simulink model "UserVehicle_RTW"  (R2022b)
settings: Solver=ode1  StartTime=0.0  StopTime=inf  FixedStep=0.001  RelTol=1e-3
PreLoadFcn:
  | vehicle = 'Car'; if ~length(which('cmself')), cmenv; end
  | UserVehicle_RTW_bus
  | UserVehicle_RTW_params
InitFcn:
  | vehicle = 'Car'; if ~length(which('cmself')), cmenv; end
  | UserVehicle_RTW_bus
values from neighbouring files (symbols this model uses):
  Car_Bdy1_mass = 650.0    (= 650)    [SingleTrack_RTW_params.m]    (also in UserVehicle_RTW_params.m)
  Car_Steering_i = 10.0    (= 10)    [SingleTrack_RTW_params.m]    (also in UserVehicle_RTW_params.m)
  Car_WhlBaseF = 1.5    [SingleTrack_RTW_params.m]    (also in UserVehicle_RTW_params.m)
  Car_WhlBaseR = -1.5    [SingleTrack_RTW_params.m]    (also in UserVehicle_RTW_params.m)
libraries: CarMaker4SL x77
(part 2 of 3)

== system UserVehicle_RTW/SingleTrack_Out/Subsystem1 ==
  In1 : Inport
  Bus Creator : BusCreator  Inputs=3
  foo_Input_Selector1 : BusSelector  OutputSignals=Vhcl v,Vhcl Distance,Vhcl sRoad,Vhcl Hitch_Pos x,Vhcl Hitch_Pos y,Vhcl Hitch_Pos z,Vhcl Roll,Vhcl RollVel,Vhcl RollAcc,Vhcl Pitch,Vhcl PitchVel,Vhcl PitchAcc,Vhcl Yaw,Vhcl YawRate,Vhcl YawAcc
  Out1 : Outport  VectorParamsAs1DForOutWhenUnconnected=off
  Out2 : Outport  Port=2  VectorParamsAs1DForOutWhenUnconnected=off
  Out3 : Outport  Port=3  VectorParamsAs1DForOutWhenUnconnected=off
  Out6 : Outport  Port=4  VectorParamsAs1DForOutWhenUnconnected=off
  Out7 : Outport  Port=5  VectorParamsAs1DForOutWhenUnconnected=off
  Out8 : Outport  Port=6  VectorParamsAs1DForOutWhenUnconnected=off
  Out9 : Outport  Port=7  VectorParamsAs1DForOutWhenUnconnected=off
  Out10 : Outport  Port=8  VectorParamsAs1DForOutWhenUnconnected=off
  Out11 : Outport  Port=9  VectorParamsAs1DForOutWhenUnconnected=off
  Out12 : Outport  Port=10  VectorParamsAs1DForOutWhenUnconnected=off
  Out13 : Outport  Port=11  VectorParamsAs1DForOutWhenUnconnected=off
  Out14 : Outport  Port=12  VectorParamsAs1DForOutWhenUnconnected=off
  Out15 : Outport  Port=13  VectorParamsAs1DForOutWhenUnconnected=off
  wires:
  foo_Input_Selector1/4 -> Bus Creator/1  "<Vhcl Hitch_Pos x>"
  foo_Input_Selector1/5 -> Bus Creator/2  "<Vhcl Hitch_Pos y>"
  foo_Input_Selector1/6 -> Bus Creator/3  "<Vhcl Hitch_Pos z>"
  foo_Input_Selector1/1 -> Out1/1  "<Vhcl v>"
  foo_Input_Selector1/2 -> Out2/1  "<Vhcl Distance>"
  foo_Input_Selector1/3 -> Out3/1  "<Vhcl sRoad>"
  Bus Creator/1 -> Out6/1
  foo_Input_Selector1/7 -> Out7/1  "<Vhcl Roll>"
  foo_Input_Selector1/8 -> Out8/1  "<Vhcl RollVel>"
  foo_Input_Selector1/9 -> Out9/1  "<Vhcl RollAcc>"
  foo_Input_Selector1/10 -> Out10/1  "<Vhcl Pitch>"
  foo_Input_Selector1/11 -> Out11/1  "<Vhcl PitchVel>"
  foo_Input_Selector1/12 -> Out12/1  "<Vhcl PitchAcc>"
  foo_Input_Selector1/13 -> Out13/1  "<Vhcl Yaw>"
  foo_Input_Selector1/14 -> Out14/1  "<Vhcl YawRate>"
  foo_Input_Selector1/15 -> Out15/1  "<Vhcl YawAcc>"
  In1/1 -> foo_Input_Selector1/1

== system UserVehicle_RTW/SingleTrack_Out/Subsystem2 ==
  In1 : Inport
  Bus Creator : BusCreator  Inputs=3
  Bus Creator1 : BusCreator  Inputs=3
  foo_Input_Selector3 : BusSelector  OutputSignals=Vhcl Wheel FL t x,Vhcl Wheel FL t y,Vhcl Wheel FL t z,Vhcl Wheel FL r_zxy x,Vhcl Wheel FL r_zxy y,Vhcl Wheel FL r_zxy z,Vhcl Wheel FL Fx,Vhcl Wheel FL Fy,Vhcl Wheel FL Fz,Vhcl Wheel FL vBelt,Vhcl Wheel FL LongSlip,Vhcl Wheel FL SideSlip,Vhcl Wheel FL Trq_T2W,Vhcl Wheel FL Trq_WhlBearing
  Out1 : Outport  VectorParamsAs1DForOutWhenUnconnected=off
  Out2 : Outport  Port=2  VectorParamsAs1DForOutWhenUnconnected=off
  Out3 : Outport  Port=3  VectorParamsAs1DForOutWhenUnconnected=off
  Out4 : Outport  Port=4  VectorParamsAs1DForOutWhenUnconnected=off
  Out5 : Outport  Port=5  VectorParamsAs1DForOutWhenUnconnected=off
  Out6 : Outport  Port=6  VectorParamsAs1DForOutWhenUnconnected=off
  Out7 : Outport  Port=7  VectorParamsAs1DForOutWhenUnconnected=off
  Out8 : Outport  Port=8  VectorParamsAs1DForOutWhenUnconnected=off
  Out9 : Outport  Port=9  VectorParamsAs1DForOutWhenUnconnected=off
  Out10 : Outport  Port=10  VectorParamsAs1DForOutWhenUnconnected=off
  wires:
  foo_Input_Selector3/1 -> Bus Creator1/1  "<Vhcl Wheel FL t x>"
  foo_Input_Selector3/2 -> Bus Creator1/2  "<Vhcl Wheel FL t y>"
  foo_Input_Selector3/3 -> Bus Creator1/3  "<Vhcl Wheel FL t z>"
  foo_Input_Selector3/4 -> Bus Creator/1  "<Vhcl Wheel FL r_zxy x>"
  foo_Input_Selector3/5 -> Bus Creator/2  "<Vhcl Wheel FL r_zxy y>"
  foo_Input_Selector3/6 -> Bus Creator/3  "<Vhcl Wheel FL r_zxy z>"
  Bus Creator1/1 -> Out1/1
  Bus Creator/1 -> Out2/1
  foo_Input_Selector3/7 -> Out3/1  "<Vhcl Wheel FL Fx>"
  In1/1 -> foo_Input_Selector3/1
  foo_Input_Selector3/8 -> Out4/1  "<Vhcl Wheel FL Fy>"
  foo_Input_Selector3/9 -> Out5/1  "<Vhcl Wheel FL Fz>"
  foo_Input_Selector3/10 -> Out6/1  "<Vhcl Wheel FL vBelt>"
  foo_Input_Selector3/11 -> Out7/1  "<Vhcl Wheel FL LongSlip>"
  foo_Input_Selector3/12 -> Out8/1  "<Vhcl Wheel FL SideSlip>"
  foo_Input_Selector3/13 -> Out9/1  "<Vhcl Wheel FL Trq_T2W>"
  foo_Input_Selector3/14 -> Out10/1  "<Vhcl Wheel FL Trq_WhlBearing>"

== system UserVehicle_RTW/SingleTrack_Out/Subsystem3 ==
  In1 : Inport
  Bus Creator : BusCreator  Inputs=3
  Bus Creator1 : BusCreator  Inputs=3
  foo_Input_Selector3 : BusSelector  OutputSignals=Vhcl Wheel FR t x,Vhcl Wheel FR t y,Vhcl Wheel FR t z,Vhcl Wheel FR r_zxy x,Vhcl Wheel FR r_zxy y,Vhcl Wheel FR r_zxy z,Vhcl Wheel FR Fx,Vhcl Wheel FR Fy,Vhcl Wheel FR Fz,Vhcl Wheel FR vBelt,Vhcl Wheel FR LongSlip,Vhcl Wheel FR SideSlip,Vhcl Wheel FR Trq_T2W,Vhcl Wheel FR Trq_WhlBearing
  Out1 : Outport  VectorParamsAs1DForOutWhenUnconnected=off
  Out2 : Outport  Port=2  VectorParamsAs1DForOutWhenUnconnected=off
  Out3 : Outport  Port=3  VectorParamsAs1DForOutWhenUnconnected=off
  Out4 : Outport  Port=4  VectorParamsAs1DForOutWhenUnconnected=off
  Out5 : Outport  Port=5  VectorParamsAs1DForOutWhenUnconnected=off
  Out6 : Outport  Port=6  VectorParamsAs1DForOutWhenUnconnected=off
  Out7 : Outport  Port=7  VectorParamsAs1DForOutWhenUnconnected=off
  Out8 : Outport  Port=8  VectorParamsAs1DForOutWhenUnconnected=off
  Out9 : Outport  Port=9  VectorParamsAs1DForOutWhenUnconnected=off
  Out10 : Outport  Port=10  VectorParamsAs1DForOutWhenUnconnected=off
  wires:
  foo_Input_Selector3/1 -> Bus Creator/1  "<Vhcl Wheel FR t x>"
  foo_Input_Selector3/2 -> Bus Creator/2  "<Vhcl Wheel FR t y>"
  foo_Input_Selector3/3 -> Bus Creator/3  "<Vhcl Wheel FR t z>"
  foo_Input_Selector3/4 -> Bus Creator1/1  "<Vhcl Wheel FR r_zxy x>"
  foo_Input_Selector3/5 -> Bus Creator1/2  "<Vhcl Wheel FR r_zxy y>"
  foo_Input_Selector3/6 -> Bus Creator1/3  "<Vhcl Wheel FR r_zxy z>"
  Bus Creator/1 -> Out1/1
  Bus Creator1/1 -> Out2/1
  foo_Input_Selector3/7 -> Out3/1  "<Vhcl Wheel FR Fx>"
  In1/1 -> foo_Input_Selector3/1
  foo_Input_Selector3/8 -> Out4/1  "<Vhcl Wheel FR Fy>"
  foo_Input_Selector3/9 -> Out5/1  "<Vhcl Wheel FR Fz>"
  foo_Input_Selector3/10 -> Out6/1  "<Vhcl Wheel FR vBelt>"
  foo_Input_Selector3/11 -> Out7/1  "<Vhcl Wheel FR LongSlip>"
  foo_Input_Selector3/12 -> Out8/1  "<Vhcl Wheel FR SideSlip>"
  foo_Input_Selector3/13 -> Out9/1  "<Vhcl Wheel FR Trq_T2W>"
  foo_Input_Selector3/14 -> Out10/1  "<Vhcl Wheel FR Trq_WhlBearing>"

== system UserVehicle_RTW/SingleTrack_Out/Subsystem4 ==
  In1 : Inport
  Bus Creator : BusCreator  Inputs=3
  Bus Creator1 : BusCreator  Inputs=3
  foo_Input_Selector3 : BusSelector  OutputSignals=Vhcl Wheel RL t x,Vhcl Wheel RL t y,Vhcl Wheel RL t z,Vhcl Wheel RL r_zxy x,Vhcl Wheel RL r_zxy y,Vhcl Wheel RL r_zxy z,Vhcl Wheel RL Fx,Vhcl Wheel RL Fy,Vhcl Wheel RL Fz,Vhcl Wheel RL vBelt,Vhcl Wheel RL LongSlip,Vhcl Wheel RL SideSlip,Vhcl Wheel RL Trq_T2W,Vhcl Wheel RL Trq_WhlBearing
  Out1 : Outport  VectorParamsAs1DForOutWhenUnconnected=off
  Out2 : Outport  Port=2  VectorParamsAs1DForOutWhenUnconnected=off
  Out3 : Outport  Port=3  VectorParamsAs1DForOutWhenUnconnected=off
  Out4 : Outport  Port=4  VectorParamsAs1DForOutWhenUnconnected=off
  Out5 : Outport  Port=5  VectorParamsAs1DForOutWhenUnconnected=off
  Out6 : Outport  Port=6  VectorParamsAs1DForOutWhenUnconnected=off
  Out7 : Outport  Port=7  VectorParamsAs1DForOutWhenUnconnected=off
  Out8 : Outport  Port=8  VectorParamsAs1DForOutWhenUnconnected=off
  Out9 : Outport  Port=9  VectorParamsAs1DForOutWhenUnconnected=off
  Out10 : Outport  Port=10  VectorParamsAs1DForOutWhenUnconnected=off
  wires:
  foo_Input_Selector3/1 -> Bus Creator/1  "<Vhcl Wheel RL t x>"
  foo_Input_Selector3/2 -> Bus Creator/2  "<Vhcl Wheel RL t y>"
  foo_Input_Selector3/3 -> Bus Creator/3  "<Vhcl Wheel RL t z>"
  foo_Input_Selector3/4 -> Bus Creator1/1  "<Vhcl Wheel RL r_zxy x>"
  foo_Input_Selector3/5 -> Bus Creator1/2  "<Vhcl Wheel RL r_zxy y>"
  foo_Input_Selector3/6 -> Bus Creator1/3  "<Vhcl Wheel RL r_zxy z>"
  Bus Creator/1 -> Out1/1
  Bus Creator1/1 -> Out2/1
  foo_Input_Selector3/7 -> Out3/1  "<Vhcl Wheel RL Fx>"
  In1/1 -> foo_Input_Selector3/1
  foo_Input_Selector3/8 -> Out4/1  "<Vhcl Wheel RL Fy>"
  foo_Input_Selector3/9 -> Out5/1  "<Vhcl Wheel RL Fz>"
  foo_Input_Selector3/10 -> Out6/1  "<Vhcl Wheel RL vBelt>"
  foo_Input_Selector3/11 -> Out7/1  "<Vhcl Wheel RL LongSlip>"
  foo_Input_Selector3/12 -> Out8/1  "<Vhcl Wheel RL SideSlip>"
  foo_Input_Selector3/13 -> Out9/1  "<Vhcl Wheel RL Trq_T2W>"
  foo_Input_Selector3/14 -> Out10/1  "<Vhcl Wheel RL Trq_WhlBearing>"

== system UserVehicle_RTW/SingleTrack_Out/Subsystem5 ==
  In1 : Inport
  Bus Creator : BusCreator  Inputs=3
  Bus Creator1 : BusCreator  Inputs=3
  foo_Input_Selector3 : BusSelector  OutputSignals=Vhcl Wheel RR t x,Vhcl Wheel RR t y,Vhcl Wheel RR t z,Vhcl Wheel RR r_zxy x,Vhcl Wheel RR r_zxy y,Vhcl Wheel RR r_zxy z,Vhcl Wheel RR Fx,Vhcl Wheel RR Fy,Vhcl Wheel RR Fz,Vhcl Wheel RR vBelt,Vhcl Wheel RR LongSlip,Vhcl Wheel RR SideSlip,Vhcl Wheel RR Trq_T2W,Vhcl Wheel RR Trq_WhlBearing
  Out1 : Outport  VectorParamsAs1DForOutWhenUnconnected=off
  Out2 : Outport  Port=2  VectorParamsAs1DForOutWhenUnconnected=off
  Out3 : Outport  Port=3  VectorParamsAs1DForOutWhenUnconnected=off
  Out4 : Outport  Port=4  VectorParamsAs1DForOutWhenUnconnected=off
  Out5 : Outport  Port=5  VectorParamsAs1DForOutWhenUnconnected=off
  Out6 : Outport  Port=6  VectorParamsAs1DForOutWhenUnconnected=off
  Out7 : Outport  Port=7  VectorParamsAs1DForOutWhenUnconnected=off
  Out8 : Outport  Port=8  VectorParamsAs1DForOutWhenUnconnected=off
  Out9 : Outport  Port=9  VectorParamsAs1DForOutWhenUnconnected=off
  Out10 : Outport  Port=10  VectorParamsAs1DForOutWhenUnconnected=off
  wires:
  foo_Input_Selector3/1 -> Bus Creator/1  "<Vhcl Wheel RR t x>"
  foo_Input_Selector3/2 -> Bus Creator/2  "<Vhcl Wheel RR t y>"
  foo_Input_Selector3/3 -> Bus Creator/3  "<Vhcl Wheel RR t z>"
  foo_Input_Selector3/4 -> Bus Creator1/1  "<Vhcl Wheel RR r_zxy x>"
  foo_Input_Selector3/5 -> Bus Creator1/2  "<Vhcl Wheel RR r_zxy y>"
  foo_Input_Selector3/6 -> Bus Creator1/3  "<Vhcl Wheel RR r_zxy z>"
  Bus Creator/1 -> Out1/1
  Bus Creator1/1 -> Out2/1
  foo_Input_Selector3/7 -> Out3/1  "<Vhcl Wheel RR Fx>"
  In1/1 -> foo_Input_Selector3/1
  foo_Input_Selector3/8 -> Out4/1  "<Vhcl Wheel RR Fy>"
  foo_Input_Selector3/9 -> Out5/1  "<Vhcl Wheel RR Fz>"
  foo_Input_Selector3/10 -> Out6/1  "<Vhcl Wheel RR vBelt>"
  foo_Input_Selector3/11 -> Out7/1  "<Vhcl Wheel RR LongSlip>"
  foo_Input_Selector3/12 -> Out8/1  "<Vhcl Wheel RR SideSlip>"
  foo_Input_Selector3/13 -> Out9/1  "<Vhcl Wheel RR Trq_T2W>"
  foo_Input_Selector3/14 -> Out10/1  "<Vhcl Wheel RR Trq_WhlBearing>"

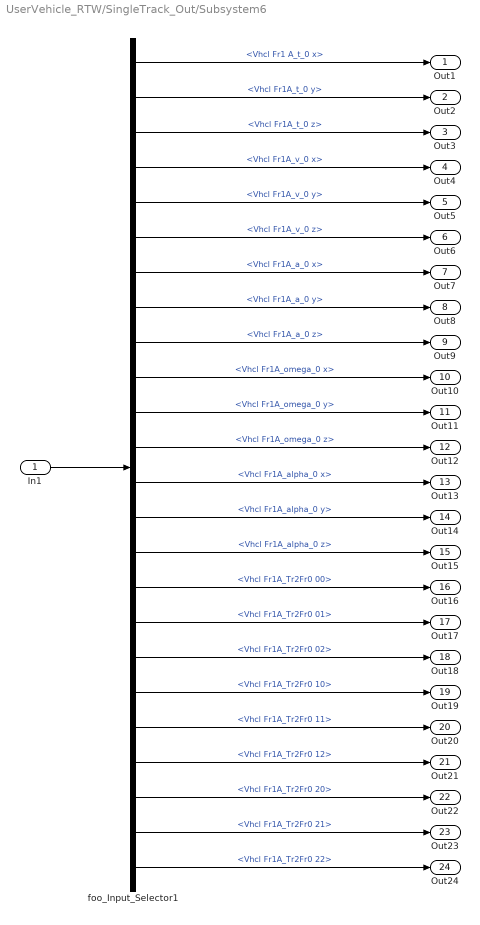
== system UserVehicle_RTW/SingleTrack_Out/Subsystem6 ==
  In1 : Inport
  foo_Input_Selector1 : BusSelector  OutputSignals=Vhcl Fr1 A_t_0 x,Vhcl Fr1A_t_0 y,Vhcl Fr1A_t_0 z,Vhcl Fr1A_v_0 x,Vhcl Fr1A_v_0 y,Vhcl Fr1A_v_0 z,Vhcl Fr1A_a_0 x,Vhcl Fr1A_a_0 y,Vhcl Fr1A_a_0 z,Vhcl Fr1A_omega_0 x,Vhcl Fr1A_omega_0 y,Vhcl Fr1A_omega_0 z,Vhcl Fr1A_alpha_0 x,Vhcl Fr1A_alpha_0 y,Vhcl Fr1A_alpha_0 z,Vhcl Fr1A_Tr2Fr0 00,Vhcl Fr1A_Tr2Fr0 01,Vhcl Fr1A_Tr2Fr0 02,Vhcl Fr1A_Tr2Fr0 10,Vhcl Fr1A_Tr2Fr0 11,Vhcl Fr1A_Tr2Fr0 12,Vhcl Fr1A_Tr2Fr0 20,Vhcl Fr1A_Tr2Fr0 21,Vhcl Fr1A_Tr2Fr0 22
  Out1 : Outport  VectorParamsAs1DForOutWhenUnconnected=off
  Out2 : Outport  Port=2  VectorParamsAs1DForOutWhenUnconnected=off
  Out3 : Outport  Port=3  VectorParamsAs1DForOutWhenUnconnected=off
  Out4 : Outport  Port=4  VectorParamsAs1DForOutWhenUnconnected=off
  Out5 : Outport  Port=5  VectorParamsAs1DForOutWhenUnconnected=off
  Out6 : Outport  Port=6  VectorParamsAs1DForOutWhenUnconnected=off
  Out7 : Outport  Port=7  VectorParamsAs1DForOutWhenUnconnected=off
  Out8 : Outport  Port=8  VectorParamsAs1DForOutWhenUnconnected=off
  Out9 : Outport  Port=9  VectorParamsAs1DForOutWhenUnconnected=off
  Out10 : Outport  Port=10  VectorParamsAs1DForOutWhenUnconnected=off
  Out11 : Outport  Port=11  VectorParamsAs1DForOutWhenUnconnected=off
  Out12 : Outport  Port=12  VectorParamsAs1DForOutWhenUnconnected=off
  Out13 : Outport  Port=13  VectorParamsAs1DForOutWhenUnconnected=off
  Out14 : Outport  Port=14  VectorParamsAs1DForOutWhenUnconnected=off
  Out15 : Outport  Port=15  VectorParamsAs1DForOutWhenUnconnected=off
  Out16 : Outport  Port=16  VectorParamsAs1DForOutWhenUnconnected=off
  Out17 : Outport  Port=17  VectorParamsAs1DForOutWhenUnconnected=off
  Out18 : Outport  Port=18  VectorParamsAs1DForOutWhenUnconnected=off
  Out19 : Outport  Port=19  VectorParamsAs1DForOutWhenUnconnected=off
  Out20 : Outport  Port=20  VectorParamsAs1DForOutWhenUnconnected=off
  Out21 : Outport  Port=21  VectorParamsAs1DForOutWhenUnconnected=off
  Out22 : Outport  Port=22  VectorParamsAs1DForOutWhenUnconnected=off
  Out23 : Outport  Port=23  VectorParamsAs1DForOutWhenUnconnected=off
  Out24 : Outport  Port=24  VectorParamsAs1DForOutWhenUnconnected=off
  wires:
  foo_Input_Selector1/24 -> Out24/1  "<Vhcl Fr1A_Tr2Fr0 22>"
  foo_Input_Selector1/23 -> Out23/1  "<Vhcl Fr1A_Tr2Fr0 21>"
  foo_Input_Selector1/22 -> Out22/1  "<Vhcl Fr1A_Tr2Fr0 20>"
  foo_Input_Selector1/21 -> Out21/1  "<Vhcl Fr1A_Tr2Fr0 12>"
  foo_Input_Selector1/20 -> Out20/1  "<Vhcl Fr1A_Tr2Fr0 11>"
  foo_Input_Selector1/19 -> Out19/1  "<Vhcl Fr1A_Tr2Fr0 10>"
  foo_Input_Selector1/18 -> Out18/1  "<Vhcl Fr1A_Tr2Fr0 02>"
  foo_Input_Selector1/17 -> Out17/1  "<Vhcl Fr1A_Tr2Fr0 01>"
  foo_Input_Selector1/16 -> Out16/1  "<Vhcl Fr1A_Tr2Fr0 00>"
  In1/1 -> foo_Input_Selector1/1
  foo_Input_Selector1/1 -> Out1/1  "<Vhcl Fr1 A_t_0 x>"
  foo_Input_Selector1/2 -> Out2/1  "<Vhcl Fr1A_t_0 y>"
  foo_Input_Selector1/3 -> Out3/1  "<Vhcl Fr1A_t_0 z>"
  foo_Input_Selector1/4 -> Out4/1  "<Vhcl Fr1A_v_0 x>"
  foo_Input_Selector1/5 -> Out5/1  "<Vhcl Fr1A_v_0 y>"
  foo_Input_Selector1/6 -> Out6/1  "<Vhcl Fr1A_v_0 z>"
  foo_Input_Selector1/7 -> Out7/1  "<Vhcl Fr1A_a_0 x>"
  foo_Input_Selector1/8 -> Out8/1  "<Vhcl Fr1A_a_0 y>"
  foo_Input_Selector1/9 -> Out9/1  "<Vhcl Fr1A_a_0 z>"
  foo_Input_Selector1/10 -> Out10/1  "<Vhcl Fr1A_omega_0 x>"
  foo_Input_Selector1/11 -> Out11/1  "<Vhcl Fr1A_omega_0 y>"
  foo_Input_Selector1/12 -> Out12/1  "<Vhcl Fr1A_omega_0 z>"
  foo_Input_Selector1/13 -> Out13/1  "<Vhcl Fr1A_alpha_0 x>"
  foo_Input_Selector1/14 -> Out14/1  "<Vhcl Fr1A_alpha_0 y>"
  foo_Input_Selector1/15 -> Out15/1  "<Vhcl Fr1A_alpha_0 z>"

== system UserVehicle_RTW/UserVehicle/CreateBus Car.Hitch.FrcTrq ==
  Bus Creator : BusCreator  Inputs=6
  Constant{1..2,7..10} (6 alike) : Constant  Value=0
  Demux7 : Demux  Outputs=6
      settings: DisplayOption=none
  Mux1 : Mux  Inputs=6
  Car.Hitch.FrcTrq : Outport  VectorParamsAs1DForOutWhenUnconnected=off
  wires:
  Demux7/1 -> Bus Creator/1  "Car Hitch Frc2Car x"
  Demux7/2 -> Bus Creator/2  "Car Hitch Frc2Car y"
  Demux7/3 -> Bus Creator/3  "Car Hitch Frc2Car z"
  Demux7/4 -> Bus Creator/4  "Car Hitch Trq2Car x"
  Demux7/5 -> Bus Creator/5  "Car Hitch Trq2Car y"
  Demux7/6 -> Bus Creator/6  "Car Hitch Trq2Car z"
  Bus Creator/1 -> Car.Hitch.FrcTrq/1
  Mux1/1 -> Demux7/1
  Constant8/1 -> Mux1/2
  Constant9/1 -> Mux1/3
  Constant10/1 -> Mux1/4
  Constant7/1 -> Mux1/1
  Constant2/1 -> Mux1/5
  Constant1/1 -> Mux1/6

== system UserVehicle_RTW/UserVehicle/CreateBus Vhcl.Fr1 ==
  Vhcl.Fr1_In : Inport
  BdyFrame2Vhcl.Fr1A : Subsystem
  Ground : Ground
  Ground1 : Ground
  Tr2Fr0 : Subsystem
  a_0 : Subsystem
  t_0 : Subsystem
  v_0 : Subsystem
  Vhcl.Fr1A : Outport  VectorParamsAs1DForOutWhenUnconnected=off
  wires:
  BdyFrame2Vhcl.Fr1A/1(Vhcl.Fr1) -> Vhcl.Fr1A/1
  Vhcl.Fr1_In/1 -> a_0/1(Car), v_0/1(Car), t_0/1(Car), Tr2Fr0/1(Car)
  Tr2Fr0/1(Tr2Fr0) -> v_0/2(Tr2Fr0), a_0/2(Tr2Fr0), BdyFrame2Vhcl.Fr1A/6(Tr2Fr0)
  t_0/1(t_0) -> BdyFrame2Vhcl.Fr1A/1(t_0)
  v_0/1(v_0) -> BdyFrame2Vhcl.Fr1A/2(v_0)
  a_0/1(a_0) -> BdyFrame2Vhcl.Fr1A/3(a_0)
  Ground1/1 -> BdyFrame2Vhcl.Fr1A/4(omega_0)
  Ground/1 -> BdyFrame2Vhcl.Fr1A/5(alpha_0)

== system UserVehicle_RTW/UserVehicle/CreateBus Vhcl.Misc ==
  In1 : Inport
  Bus Creator5 : BusCreator  Inputs=11
  Demux5 : Demux  Outputs=11
      settings: DisplayOption=none
  Out1 : Outport  VectorParamsAs1DForOutWhenUnconnected=off
  wires:
  Demux5/1 -> Bus Creator5/1  "Vhcl Trq_DL2Bdy1 x"
  Demux5/2 -> Bus Creator5/2  "Vhcl Trq_DL2Bdy1 y"
  Bus Creator5/1 -> Out1/1
  In1/1 -> Demux5/1
  Demux5/3 -> Bus Creator5/3  "Vhcl Trq_DL2Bdy1 z"
  Demux5/4 -> Bus Creator5/4  "Vhcl TrqDL2Bdy1B x"
  Demux5/5 -> Bus Creator5/5  "Vhcl TrqDL2Bdy1B y"
  Demux5/6 -> Bus Creator5/6  "Vhcl TrqDL2Bdy1B z"
  Demux5/7 -> Bus Creator5/7  "Vhcl DL2BdyEng x"
  Demux5/8 -> Bus Creator5/8  "Vhcl DL2BdyEng y"
  Demux5/9 -> Bus Creator5/9  "Vhcl Wind_vel_0 x"
  Demux5/10 -> Bus Creator5/10  "Vhcl Wind_vel_0 y"
  Demux5/11 -> Bus Creator5/11  "Vhcl Wind_vel_0 z"

== system UserVehicle_RTW/UserVehicle/CreateBus Vhcl.Motion ==
  Vhcl_Motion_In : Inport
  Bus Creator : BusCreator  Inputs=16
  Bus Selector : BusSelector  OutputSignals=Car_v_1.Car_vx_1,Car_Dist,Car_sRoad,Road_Fr1_rx,Road_Fr1_ry,Car_Yaw.Yaw,Car_Yaw.Yawp,Car_Yaw.Yawpp
  Constant{2..4,6..7,9..10} (7 alike) : Constant  Value=0
  Demux1 : Demux  Outputs=16
      settings: DisplayOption=none
  Mux1 : Mux  Inputs=16
  Vhcl.Motion : Outport  VectorParamsAs1DForOutWhenUnconnected=off
  wires:
  Vhcl_Motion_In/1 -> Bus Selector/1
  Demux1/16 -> Bus Creator/16  "Vhcl YawAcc"
  Demux1/15 -> Bus Creator/15  "Vhcl YawRate"
  Demux1/14 -> Bus Creator/14  "Vhcl Yaw"
  Demux1/13 -> Bus Creator/13  "Vhcl PitchAcc"
  Demux1/12 -> Bus Creator/12  "Vhcl PitchVel"
  Demux1/11 -> Bus Creator/11  "Vhcl Pitch"
  Demux1/10 -> Bus Creator/10  "Vhcl RollAcc"
  Demux1/9 -> Bus Creator/9  "Vhcl RollVel"
  Demux1/8 -> Bus Creator/8  "Vhcl Roll"
  Demux1/7 -> Bus Creator/7  "Vhcl Hitch_Pos z"
  Demux1/6 -> Bus Creator/6  "Vhcl Hitch_Pos y"
  Demux1/5 -> Bus Creator/5  "Vhcl Hitch_Pos x"
  Demux1/4 -> Bus Creator/4  "Vhcl sRoadAero"
  Demux1/3 -> Bus Creator/3  "Vhcl sRoad"
  Demux1/2 -> Bus Creator/2  "Vhcl Distance"
  Demux1/1 -> Bus Creator/1  "Vhcl v"
  Bus Creator/1 -> Vhcl.Motion/1
  Mux1/1 -> Demux1/1
  Bus Selector/1 -> Mux1/1  "<Car_vx_1>"
  Bus Selector/2 -> Mux1/2  "<Car_Dist>"
  Constant2/1 -> Mux1/5
  Constant3/1 -> Mux1/6
  Constant4/1 -> Mux1/7
  Constant6/1 -> Mux1/9
  Constant7/1 -> Mux1/10
  Constant9/1 -> Mux1/12
  Constant10/1 -> Mux1/13
  Bus Selector/6 -> Mux1/14  "<Yaw>"
  Bus Selector/7 -> Mux1/15  "<Yawp>"
  Bus Selector/8 -> Mux1/16  "<Yawpp>"
  Bus Selector/4 -> Mux1/8  "<Road_Fr1_rx>"
  Bus Selector/5 -> Mux1/11  "<Road_Fr1_ry>"
  Bus Selector/3 -> Mux1/4, Mux1/3  "<Car_sRoad>"

== system UserVehicle_RTW/UserVehicle/CreateBus Vhcl.PT ==
  In1 : Inport
  Bus Creator3 : BusCreator  Inputs=6
  Demux3 : Demux  Outputs=6
      settings: DisplayOption=none
  Out1 : Outport  VectorParamsAs1DForOutWhenUnconnected=off
  wires:
  Demux3/6 -> Bus Creator3/6  "VhclCtrl Gas"
  Demux3/3 -> Bus Creator3/3  "VhclCtrl StarterCtrl"
  Demux3/5 -> Bus Creator3/5  "VhclCtrl SelectorManualShift"
  Demux3/1 -> Bus Creator3/1  "VhclCtrl Key"
  Demux3/2 -> Bus Creator3/2  "VhclCtrl SST"
  Demux3/4 -> Bus Creator3/4  "VhclCtrl SelectorCtrl"
  Bus Creator3/1 -> Out1/1
  In1/1 -> Demux3/1

== system UserVehicle_RTW/UserVehicle/CreateBus Vhcl.PoI ==
  Vhcl_POI_In : Inport
  Bus Creator : BusCreator  Inputs=18
  Bus Selector : BusSelector  OutputSignals=Car_t_0.Car_tx_0,Car_t_0.Car_ty_0,Road_Fr1_z,Car_v_0.Car_vx_0,Car_v_0.Car_vy_0,Car_a_0.Car_ax_0,Car_a_0.Car_ay_0,Car_v_1.Car_vx_1,Car_v_1.Car_vy_1,Car_a_1.Car_ax_1,Car_a_1.Car_ay_1
  Constant{11..13,15..16,18..19} (7 alike) : Constant  Value=0
  Demux3 : Demux  Outputs=18
      settings: DisplayOption=none
  Mux1 : Mux  Inputs=18
  Vhcl.PoI : Outport  VectorParamsAs1DForOutWhenUnconnected=off
  wires:
  Bus Selector/9 -> Mux1/11  "<Car_vy_1>"
  Demux3/1 -> Bus Creator/1  "Vhcl PoI_Pos x"
  Bus Creator/1 -> Vhcl.PoI/1
  Demux3/2 -> Bus Creator/2  "Vhcl PoI_Pos y"
  Demux3/3 -> Bus Creator/3  "Vhcl PoI_Pos z"
  Demux3/4 -> Bus Creator/4  "Vhcl PoI_Vel x"
  Demux3/5 -> Bus Creator/5  "Vhcl PoI_Vel y"
  Demux3/6 -> Bus Creator/6  "Vhcl PoI_Vel z"
  Demux3/7 -> Bus Creator/7  "Vhcl PoI_Acc x"
  Demux3/8 -> Bus Creator/8  "Vhcl PoI_Acc y"
  Demux3/9 -> Bus Creator/9  "Vhcl PoI_Acc z"
  Demux3/10 -> Bus Creator/10  "Vhcl PoI_Vel_1 x"
  Demux3/11 -> Bus Creator/11  "Vhcl PoI_Vel_1 y"
  Demux3/12 -> Bus Creator/12  "Vhcl PoI_Vel_1 z"
  Demux3/13 -> Bus Creator/13  "Vhcl PoI_Acc_1 x"
  Demux3/14 -> Bus Creator/14  "Vhcl PoI_Acc_1 y"
  Demux3/15 -> Bus Creator/15  "Vhcl PoI_Acc_1 z"
  Demux3/16 -> Bus Creator/16  "Vhcl PoI_GCS Long"
  Demux3/17 -> Bus Creator/17  "Vhcl PoI_GCS Lat"
  Demux3/18 -> Bus Creator/18  "Vhcl PoI_GCS Elev"
  Mux1/1 -> Demux3/1
  Vhcl_POI_In/1 -> Bus Selector/1
  Constant12/1 -> Mux1/16
  Constant13/1 -> Mux1/17
  Constant11/1 -> Mux1/18
  Bus Selector/1 -> Mux1/1  "<Car_tx_0>"
  Bus Selector/2 -> Mux1/2  "<Car_ty_0>"
  Bus Selector/3 -> Mux1/3  "<Road_Fr1_z>"
  Bus Selector/4 -> Mux1/4  "<Car_vx_0>"
  Bus Selector/5 -> Mux1/5  "<Car_vy_0>"
  Constant15/1 -> Mux1/6
  Bus Selector/6 -> Mux1/7  "<Car_ax_0>"
  Constant16/1 -> Mux1/9
  Constant18/1 -> Mux1/12
  Bus Selector/10 -> Mux1/13  "<Car_ax_1>"
  Bus Selector/11 -> Mux1/14  "<Car_ay_1>"
  Constant19/1 -> Mux1/15
  Bus Selector/7 -> Mux1/8  "<Car_ay_0>"
  Bus Selector/8 -> Mux1/10  "<Car_vx_1>"

== system UserVehicle_RTW/UserVehicle/CreateBus Vhcl.Steering ==
  Vhcl_Steering_In : Inport
  Bus Creator : BusCreator  Inputs=4
  Bus Selector : BusSelector  OutputSignals=VhclCtrl Steering Ang,VhclCtrl Steering AngVel,VhclCtrl Steering AngAcc,VhclCtrl Steering Trq
  Demux : Demux
      settings: DisplayOption=none
  Mux1 : Mux
  Vhcl.Steering : Outport  VectorParamsAs1DForOutWhenUnconnected=off
  wires:
  Demux/4 -> Bus Creator/4  "Vhcl Steering Trq"
  Demux/2 -> Bus Creator/2  "Vhcl Steering AngVel"
  Demux/3 -> Bus Creator/3  "Vhcl Steering AngAcc"
  Demux/1 -> Bus Creator/1  "Vhcl Steering Ang"
  Bus Creator/1 -> Vhcl.Steering/1
  Vhcl_Steering_In/1 -> Bus Selector/1
  Bus Selector/1 -> Mux1/1  "<VhclCtrl Steering Ang>"
  Bus Selector/2 -> Mux1/2  "<VhclCtrl Steering AngVel>"
  Bus Selector/3 -> Mux1/3  "<VhclCtrl Steering AngAcc>"
  Bus Selector/4 -> Mux1/4  "<VhclCtrl Steering Trq>"
  Mux1/1 -> Demux/1

== system UserVehicle_RTW/UserVehicle/CreateBus Vhcl.Wheel.FL ==
  Vhcl.Wheel.FL_In : Inport
  Bus Creator : BusCreator  Inputs=14
  Bus Selector : BusSelector  OutputSignals=Car_Whl_F_rz,Car_Tire.Car_Tire_F.LongFrc,Car_Tire.Car_Tire_F.SideFrc,Car_Whl_F_1.Car_F_Fz_1,Car_Tire.Car_Tire_F.vBelt,Car_Tire.Car_Tire_F.Slp,Car_Tire.Car_Tire_F.Alpha,Car_Trq2W.Trq_F
  Constant{1..5,11} (6 alike) : Constant  Value=0
  Demux3 : Demux  Outputs=14
      settings: DisplayOption=none
  Mux1 : Mux  Inputs=14
  Vhcl.Wheel.FL : Outport  VectorParamsAs1DForOutWhenUnconnected=off
  wires:
  Bus Selector/7 -> Mux1/12  "<Alpha>"
  Bus Selector/5 -> Mux1/10  "<vBelt>"
  Demux3/1 -> Bus Creator/1  "Vhcl Wheel FL t x"
  Bus Creator/1 -> Vhcl.Wheel.FL/1
  Mux1/1 -> Demux3/1
  Demux3/2 -> Bus Creator/2  "Vhcl Wheel FL t y"
  Demux3/3 -> Bus Creator/3  "Vhcl Wheel FL t z"
  Demux3/4 -> Bus Creator/4  "Vhcl Wheel FL r_zxy x"
  Demux3/5 -> Bus Creator/5  "Vhcl Wheel FL r_zxy y"
  Demux3/6 -> Bus Creator/6  "Vhcl Wheel FL r_zxy z"
  Demux3/7 -> Bus Creator/7  "Vhcl Wheel FL Fx"
  Demux3/8 -> Bus Creator/8  "Vhcl Wheel FL Fy"
  Demux3/9 -> Bus Creator/9  "Vhcl Wheel FL Fz"
  Demux3/10 -> Bus Creator/10  "Vhcl Wheel FL vBelt"
  Demux3/11 -> Bus Creator/11  "Vhcl Wheel FL LongSlip"
  Demux3/12 -> Bus Creator/12  "Vhcl Wheel FL SideSlip"
  Demux3/13 -> Bus Creator/13  "Vhcl Wheel FL Trq_T2W"
  Demux3/14 -> Bus Creator/14  "Vhcl Wheel FL Trq_WhlBearing"
  Vhcl.Wheel.FL_In/1 -> Bus Selector/1
  Bus Selector/1 -> Mux1/6  "<Car_Whl_F_rz>"
  Constant1/1 -> Mux1/1
  Constant2/1 -> Mux1/2
  Constant3/1 -> Mux1/3
  Constant4/1 -> Mux1/4
  Constant5/1 -> Mux1/5
  Bus Selector/2 -> Mux1/7  "<LongFrc>"
  Bus Selector/3 -> Mux1/8  "<SideFrc>"
  Bus Selector/6 -> Mux1/11  "<Slp>"
  Bus Selector/8 -> Mux1/13  "<Trq_F>"
  Constant11/1 -> Mux1/14
  Bus Selector/4 -> Mux1/9  "<Car_F_Fz_1>"

== system UserVehicle_RTW/UserVehicle/CreateBus Vhcl.Wheel.FR ==
  Vhcl.Wheel.FR_In : Inport
  Bus Creator : BusCreator  Inputs=14
  Bus Selector : BusSelector  OutputSignals=Car_Whl_F_rz,Car_Tire.Car_Tire_F.LongFrc,Car_Tire.Car_Tire_F.SideFrc,Car_Whl_F_1.Car_F_Fz_1,Car_Tire.Car_Tire_F.vBelt,Car_Tire.Car_Tire_F.Slp,Car_Tire.Car_Tire_F.Alpha,Car_Trq2W.Trq_F
  Constant{1..5,11} (6 alike) : Constant  Value=0
  Demux3 : Demux  Outputs=14
      settings: DisplayOption=none
  Mux1 : Mux  Inputs=14
  Vhcl.Wheel.FR : Outport  VectorParamsAs1DForOutWhenUnconnected=off
  wires:
  Demux3/1 -> Bus Creator/1  "Vhcl Wheel FR t x"
  Bus Creator/1 -> Vhcl.Wheel.FR/1
  Demux3/2 -> Bus Creator/2  "Vhcl Wheel FR t y"
  Demux3/3 -> Bus Creator/3  "Vhcl Wheel FR t z"
  Demux3/4 -> Bus Creator/4  "Vhcl Wheel FR r_zxy x"
  Demux3/5 -> Bus Creator/5  "Vhcl Wheel FR r_zxy y"
  Demux3/6 -> Bus Creator/6  "Vhcl Wheel FR r_zxy z"
  Demux3/7 -> Bus Creator/7  "Vhcl Wheel FR Fx"
  Demux3/8 -> Bus Creator/8  "Vhcl Wheel FR Fy"
  Demux3/9 -> Bus Creator/9  "Vhcl Wheel FR Fz"
  Demux3/10 -> Bus Creator/10  "Vhcl Wheel FR vBelt"
  Demux3/11 -> Bus Creator/11  "Vhcl Wheel FR LongSlip"
  Demux3/12 -> Bus Creator/12  "Vhcl Wheel FR SideSlip"
  Demux3/13 -> Bus Creator/13  "Vhcl Wheel FR Trq_T2W"
  Demux3/14 -> Bus Creator/14  "Vhcl Wheel FR Trq_WhlBearing"
  Mux1/1 -> Demux3/1
  Vhcl.Wheel.FR_In/1 -> Bus Selector/1
  Bus Selector/1 -> Mux1/6  "<Car_Whl_F_rz>"
  Constant1/1 -> Mux1/1
  Constant2/1 -> Mux1/2
  Constant3/1 -> Mux1/3
  Constant4/1 -> Mux1/4
  Constant5/1 -> Mux1/5
  Bus Selector/2 -> Mux1/7  "<LongFrc>"
  Bus Selector/3 -> Mux1/8  "<SideFrc>"
  Bus Selector/4 -> Mux1/9  "<Car_F_Fz_1>"
  Bus Selector/7 -> Mux1/12  "<Alpha>"
  Bus Selector/5 -> Mux1/10  "<vBelt>"
  Bus Selector/6 -> Mux1/11  "<Slp>"
  Bus Selector/8 -> Mux1/13  "<Trq_F>"
  Constant11/1 -> Mux1/14

== system UserVehicle_RTW/UserVehicle/CreateBus Vhcl.Wheel.In ==
  In1 : Inport
  Bus Creator1 : BusCreator  Inputs=12
  Demux1 : Demux  Outputs=12
      settings: DisplayOption=none
  Out1 : Outport  VectorParamsAs1DForOutWhenUnconnected=off
  wires:
  Demux1/1 -> Bus Creator1/1  "Vhcl Wheel FL Trq_B2WC"
  Demux1/2 -> Bus Creator1/2  "Vhcl Wheel FL Trq_DL2WC"
  Bus Creator1/1 -> Out1/1
  In1/1 -> Demux1/1
  Demux1/3 -> Bus Creator1/3  "Vhcl Wheel FL rotv"
  Demux1/4 -> Bus Creator1/4  "Vhcl Wheel FR Trq_B2WC"
  Demux1/5 -> Bus Creator1/5  "Vhcl Wheel FR Trq_DL2WC"
  Demux1/6 -> Bus Creator1/6  "Vhcl Wheel FR rotv"
  Demux1/7 -> Bus Creator1/7  "Vhcl Wheel RL Trq_B2WC"
  Demux1/8 -> Bus Creator1/8  "Vhcl Wheel RL Trq_DL2WC"
  Demux1/9 -> Bus Creator1/9  "Vhcl Wheel RL rotv"
  Demux1/10 -> Bus Creator1/10  "Vhcl Wheel RR Trq_B2WC"
  Demux1/11 -> Bus Creator1/11  "Vhcl Wheel RR Trq_DL2WC"
  Demux1/12 -> Bus Creator1/12  "Vhcl Wheel RR rotv"

== system UserVehicle_RTW/UserVehicle/CreateBus Vhcl.Wheel.RL ==
  Vhcl.Wheel.RL_In : Inport
  Bus Creator : BusCreator  Inputs=14
  Bus Selector : BusSelector  OutputSignals=Car_Tire.Car_Tire_R.LongFrc,Car_Tire.Car_Tire_R.SideFrc,Car_Whl_F_1.Car_R_Fz_1,Car_Tire.Car_Tire_R.vBelt,Car_Tire.Car_Tire_R.Slp,Car_Tire.Car_Tire_R.Alpha,Car_Trq2W.Trq_R
  Constant{1..5,11,13} (7 alike) : Constant  Value=0
  Demux3 : Demux  Outputs=14
      settings: DisplayOption=none
  Mux1 : Mux  Inputs=14
  Vhcl.Wheel.RL : Outport  VectorParamsAs1DForOutWhenUnconnected=off
  wires:
  Demux3/1 -> Bus Creator/1  "Vhcl Wheel RL t x"
  Bus Creator/1 -> Vhcl.Wheel.RL/1
  Demux3/2 -> Bus Creator/2  "Vhcl Wheel RL t y"
  Demux3/3 -> Bus Creator/3  "Vhcl Wheel RL t z"
  Demux3/4 -> Bus Creator/4  "Vhcl Wheel RL r_zxy x"
  Demux3/5 -> Bus Creator/5  "Vhcl Wheel RL r_zxy y"
  Demux3/6 -> Bus Creator/6  "Vhcl Wheel RL r_zxy z"
  Demux3/7 -> Bus Creator/7  "Vhcl Wheel RL Fx"
  Demux3/8 -> Bus Creator/8  "Vhcl Wheel RL Fy"
  Demux3/9 -> Bus Creator/9  "Vhcl Wheel RL Fz"
  Demux3/10 -> Bus Creator/10  "Vhcl Wheel RL vBelt"
  Demux3/11 -> Bus Creator/11  "Vhcl Wheel RL LongSlip"
  Demux3/12 -> Bus Creator/12  "Vhcl Wheel RL SideSlip"
  Demux3/13 -> Bus Creator/13  "Vhcl Wheel RL Trq_T2W"
  Demux3/14 -> Bus Creator/14  "Vhcl Wheel RL Trq_WhlBearing"
  Mux1/1 -> Demux3/1
  Vhcl.Wheel.RL_In/1 -> Bus Selector/1
  Constant1/1 -> Mux1/1
  Constant2/1 -> Mux1/2
  Constant3/1 -> Mux1/3
  Constant4/1 -> Mux1/4
  Constant5/1 -> Mux1/5
  Bus Selector/1 -> Mux1/7  "<LongFrc>"
  Bus Selector/2 -> Mux1/8  "<SideFrc>"
  Bus Selector/3 -> Mux1/9  "<Car_R_Fz_1>"
  Bus Selector/7 -> Mux1/13  "<Trq_R>"
  Constant11/1 -> Mux1/14
  Constant13/1 -> Mux1/6
  Bus Selector/6 -> Mux1/12  "<Alpha>"
  Bus Selector/4 -> Mux1/10  "<vBelt>"
  Bus Selector/5 -> Mux1/11  "<Slp>"

== system UserVehicle_RTW/UserVehicle/CreateBus Vhcl.Wheel.RR ==
  Vhcl.Wheel.RR_In : Inport
  Bus Creator : BusCreator  Inputs=14
  Bus Selector : BusSelector  OutputSignals=Car_Tire.Car_Tire_R.LongFrc,Car_Tire.Car_Tire_R.SideFrc,Car_Whl_F_1.Car_R_Fz_1,Car_Tire.Car_Tire_R.vBelt,Car_Tire.Car_Tire_R.Slp,Car_Tire.Car_Tire_R.Alpha,Car_Trq2W.Trq_R
  Constant{1..5,11,13} (7 alike) : Constant  Value=0
  Demux3 : Demux  Outputs=14
      settings: DisplayOption=none
  Mux1 : Mux  Inputs=14
  Vhcl.Wheel.RR : Outport  VectorParamsAs1DForOutWhenUnconnected=off
  wires:
  Bus Creator/1 -> Vhcl.Wheel.RR/1
  Bus Selector/1 -> Mux1/7  "<LongFrc>"
  Demux3/1 -> Bus Creator/1  "Vhcl Wheel RR t x"
  Demux3/2 -> Bus Creator/2  "Vhcl Wheel RR t y"
  Demux3/3 -> Bus Creator/3  "Vhcl Wheel RR t z"
  Demux3/4 -> Bus Creator/4  "Vhcl Wheel RR r_zxy x"
  Demux3/5 -> Bus Creator/5  "Vhcl Wheel RR r_zxy y"
  Demux3/6 -> Bus Creator/6  "Vhcl Wheel RR r_zxy z"
  Demux3/7 -> Bus Creator/7  "Vhcl Wheel RR Fx"
  Demux3/8 -> Bus Creator/8  "Vhcl Wheel RR Fy"
  Demux3/9 -> Bus Creator/9  "Vhcl Wheel RR Fz"
  Demux3/10 -> Bus Creator/10  "Vhcl Wheel RR vBelt"
  Demux3/11 -> Bus Creator/11  "Vhcl Wheel RR LongSlip"
  Demux3/12 -> Bus Creator/12  "Vhcl Wheel RR SideSlip"
  Demux3/13 -> Bus Creator/13  "Vhcl Wheel RR Trq_T2W"
  Demux3/14 -> Bus Creator/14  "Vhcl Wheel RR Trq_WhlBearing"
  Mux1/1 -> Demux3/1
  Vhcl.Wheel.RR_In/1 -> Bus Selector/1
  Constant1/1 -> Mux1/1
  Constant2/1 -> Mux1/2
  Constant3/1 -> Mux1/3
  Constant4/1 -> Mux1/4
  Constant5/1 -> Mux1/5
  Bus Selector/2 -> Mux1/8  "<SideFrc>"
  Bus Selector/3 -> Mux1/9  "<Car_R_Fz_1>"
  Bus Selector/7 -> Mux1/13  "<Trq_R>"
  Constant11/1 -> Mux1/14
  Constant13/1 -> Mux1/6
  Bus Selector/6 -> Mux1/12  "<Alpha>"
  Bus Selector/4 -> Mux1/10  "<vBelt>"
  Bus Selector/5 -> Mux1/11  "<Slp>"

== system UserVehicle_RTW/UserVehicle/CreateBus VhclCtrl.Steering ==
  In1 : Inport
  Bus Creator : BusCreator  Inputs=5
  Demux : Demux  Outputs=5
      settings: DisplayOption=none
  Out1 : Outport  VectorParamsAs1DForOutWhenUnconnected=off
  wires:
  Demux/4 -> Bus Creator/4  "VhclCtrl Steering Trq"
  Demux/2 -> Bus Creator/2  "VhclCtrl Steering AngVel"
  Demux/3 -> Bus Creator/3  "VhclCtrl Steering AngAcc"
  Demux/5 -> Bus Creator/5  "VhclCtrl Steering ByTrq"
  Demux/1 -> Bus Creator/1  "VhclCtrl Steering Ang"
  Bus Creator/1 -> Out1/1
  In1/1 -> Demux/1

== system UserVehicle_RTW/UserVehicle/Query Road CoG ==
  In1 : Inport
  Bus Selector1 : BusSelector  OutputSignals=Car_t_0.Car_tx_0,Car_t_0.Car_ty_0,Car_Dist
  Bus Selector2 : BusSelector  OutputSignals=z,slope,grade,s
  Constant1 : Constant  Value=0
  Constant2 : Constant  Value=0
  Mux : Mux  Inputs=3
  Read CM Parameter : CarMaker4SL/Read CM Parameter  xfile_type=Vehicle  xfile_instance_vehicle=-  xfile_instance_trailer=1  xfile_instance_general=-  xfile_kind_vehicle=Vehicle  xfile_kind_trailer=Trailer  xfile_kind_general=SimParameters  xfile=Vehicle  xkey=Wheel.fl.pos  xnout=1  xdefaults=0  xmuxed=on  xstime=Continuous
      settings: SourceProductName=CarMaker4SL
  Subsystem : Subsystem
  Sum2 : Sum  InputSameDT=on  SaturateOnIntegerOverflow=on  OutDataTypeStr=Inherit: Same as first input
  neg : Gain  Gain=-1  SaturateOnIntegerOverflow=on  OutDataTypeStr=Inherit: Same as input  ParamDataTypeStr=Inherit: Same as input
  Fr1_z : Outport  VectorParamsAs1DForOutWhenUnconnected=off
  Fr1_rx : Outport  Port=2  VectorParamsAs1DForOutWhenUnconnected=off
  Fr1_ry : Outport  Port=3  VectorParamsAs1DForOutWhenUnconnected=off
  sRoad : Outport  Port=4  VectorParamsAs1DForOutWhenUnconnected=off
  wires:
  [TRSim] -> Subsystem/Enable
  Constant2/1 -> Mux/3
  Bus Selector2/2 -> Fr1_rx/1  "<slope>"
  Bus Selector2/1 -> Fr1_z/1  "<z>"
  In1/1 -> Bus Selector1/1
  Bus Selector1/3 -> Subsystem/2(Dist)  "<Car_Dist>"
  Mux/1 -> Subsystem/1(xyz)
  Bus Selector1/2 -> Mux/2  "<Car_ty_0>"
  Bus Selector1/1 -> Mux/1  "<Car_tx_0>"
  Subsystem/1(Tire) -> Bus Selector2/1
  Constant1/1 -> Subsystem/3(Side)
  Bus Selector2/3 -> neg/1  "<grade>"
  neg/1 -> Fr1_ry/1
  Bus Selector2/4 -> Sum2/1  "<s>"
  Sum2/1 -> sRoad/1
  Read CM Parameter/1 -> Sum2/2

== system UserVehicle_RTW/UserVehicle/SimStates ==
  note: Detect CarMaker states and transistions relevant for initialization at the start of a new Test Run.
  Logical Operator : Logic  AllPortsSameDT=off  OutDataTypeStr=boolean
  Logical Operator1 : Logic  Operator=OR  AllPortsSameDT=off  OutDataTypeStr=boolean
  Memory : Memory
  Read CM Dict : CarMaker4SL/Read CM Dict  xname=SC.State  xsync=off  xstime=Continuous
  Read CM Dict1 : CarMaker4SL/Read CM Dict  xname=Time  xsync=off  xstime=Continuous
  Relational Operator : RelationalOperator  Operator=<=  OutDataTypeStr=boolean  InputSameDT=off
  Relational Operator1 : RelationalOperator  Operator===  OutDataTypeStr=boolean  InputSameDT=off
  Relational Operator2 : RelationalOperator  Operator===  OutDataTypeStr=boolean  InputSameDT=off
  SCState_Simulate : Constant  Value=8
  Zero : Constant  Value=0
  detect increase : RelationalOperator  Operator=>  OutDataTypeStr=boolean  InputSameDT=off
  tag scope: TRSim=global, TRStart=global
  wires:
  Read CM Dict/1 -> Relational Operator/1, Relational Operator1/2, Memory/1, detect increase/1
  SCState_Simulate/1 -> Relational Operator/2, Relational Operator1/1
  Relational Operator/1 -> Logical Operator/2
  Read CM Dict1/1 -> Relational Operator2/1
  Zero/1 -> Relational Operator2/2
  Relational Operator2/1 -> Logical Operator1/1
  Logical Operator/1 -> Logical Operator1/2
  Logical Operator1/1 -> [TRStart]
  detect increase/1 -> Logical Operator/1
  Memory/1 -> detect increase/2
  Relational Operator1/1 -> [TRSim]

== system UserVehicle_RTW/UserVehicle/Single Track Model ==
  note: Formeln nach:
      | Schramm, Hiller, Bardini
      | Modellbildung und Simulation der Dynamik von Kraftfahrzeugen
      | Seite 244 ff
      | ISBN 978-3-540-89313-4
  VhclCtrl.Steering : Inport
  Vhcl.Wheel.In : Inport  Port=2
  Tire2Wheel : Subsystem
  sideslip angle : Subsystem
  steer kinematic : Subsystem
  tire forces : Subsystem
  vehicle motion : Subsystem
  wheel torques : Subsystem
  yaw : Subsystem
  Car.a_1 : Outport  VectorParamsAs1DForOutWhenUnconnected=off
  Car.v_1 : Outport  Port=2  VectorParamsAs1DForOutWhenUnconnected=off
  Car.a_0 : Outport  Port=3  VectorParamsAs1DForOutWhenUnconnected=off
  Car.v_0 : Outport  Port=4  VectorParamsAs1DForOutWhenUnconnected=off
  Car.t_0 : Outport  Port=5  VectorParamsAs1DForOutWhenUnconnected=off
  Car.Dist : Outport  Port=6  VectorParamsAs1DForOutWhenUnconnected=off
  Car.Yaw : Outport  Port=7  VectorParamsAs1DForOutWhenUnconnected=off
  Car.Tire : Outport  Port=8  VectorParamsAs1DForOutWhenUnconnected=off
  Car.Trq2W : Outport  Port=9  VectorParamsAs1DForOutWhenUnconnected=off
  Car.Whl.F.rz : Outport  Port=10  VectorParamsAs1DForOutWhenUnconnected=off
  Car.Whl.F_1 : Outport  Port=11  VectorParamsAs1DForOutWhenUnconnected=off
  wires:
  Tire2Wheel/1(Car.Whl.F_1) -> vehicle motion/1(Car.Whl.F_1), tire forces/7(Car.Whl.F_1), Car.Whl.F_1/1, yaw/1(WheelFrc_1)
  tire forces/1(Tire) -> wheel torques/1(WheelTrq_1), Car.Tire/1, Tire2Wheel/1(Tire)
  Vhcl.Wheel.In/1 -> tire forces/5(Vhcl.Wheel.In)
  vehicle motion/5(Car_t_0) -> tire forces/4(Car_t_0), Car.t_0/1
  vehicle motion/4(Car.v_0) -> Car.v_0/1
  vehicle motion/3(Car.a_0) -> Car.a_0/1
  vehicle motion/6(Car.Dist) -> Car.Dist/1
  vehicle motion/1(Car.a_1) -> sideslip angle/1(Car_a_1), Car.a_1/1
  sideslip angle/1(beta) -> vehicle motion/2(Car.Beta), tire forces/2(beta)  "beta"
  vehicle motion/2(Car.v_1) -> sideslip angle/2(Car_v_1), Car.v_1/1, tire forces/3(Car_v_1)
  steer kinematic/1(Car.Whl.F.rz) -> Tire2Wheel/2(Wheel_rz), tire forces/6(Car.Wheel.rz), Car.Whl.F.rz/1
  VhclCtrl.Steering/1 -> steer kinematic/1(In1)
  wheel torques/1(Car.Trq2W) -> Car.Trq2W/1
  yaw/1(Car.Yaw) -> vehicle motion/3(Car_Yaw), sideslip angle/3(Yaw), tire forces/1(Yaw), Car.Yaw/1

== system UserVehicle_RTW/UserVehicle/CreateBus Vhcl.Fr1/BdyFrame2Vhcl.Fr1A ==
  note: Translate pseudo BdyFrame interface to Vhcl.Fr1
  t_0 : Inport
  v_0 : Inport  Port=2
  a_0 : Inport  Port=3
  omega_0 : Inport  Port=4
  alpha_0 : Inport  Port=5
  Tr2Fr0 : Inport  Port=6
  Bus Creator : BusCreator  Inputs=24
  Demux{,1..3,5} (5 alike) : Demux  Outputs=3
  Demux4 : Demux  Outputs=9
  Vhcl.Fr1 : Outport  VectorParamsAs1DForOutWhenUnconnected=off
  wires:
  Bus Creator/1 -> Vhcl.Fr1/1
  Demux/1 -> Bus Creator/1  "Vhcl Fr1 A_t_0 x"
  Demux/2 -> Bus Creator/2  "Vhcl Fr1A_t_0 y"
  Demux/3 -> Bus Creator/3  "Vhcl Fr1A_t_0 z"
  Demux1/1 -> Bus Creator/4  "Vhcl Fr1A_v_0 x"
  Demux1/2 -> Bus Creator/5  "Vhcl Fr1A_v_0 y"
  Demux1/3 -> Bus Creator/6  "Vhcl Fr1A_v_0 z"
  Demux2/1 -> Bus Creator/7  "Vhcl Fr1A_a_0 x"
  Demux2/2 -> Bus Creator/8  "Vhcl Fr1A_a_0 y"
  Demux2/3 -> Bus Creator/9  "Vhcl Fr1A_a_0 z"
  Demux3/1 -> Bus Creator/10  "Vhcl Fr1A_omega_0 x"
  Demux3/2 -> Bus Creator/11  "Vhcl Fr1A_omega_0 y"
  Demux3/3 -> Bus Creator/12  "Vhcl Fr1A_omega_0 z"
  Demux5/1 -> Bus Creator/13  "Vhcl Fr1A_alpha_0 x"
  Demux5/2 -> Bus Creator/14  "Vhcl Fr1A_alpha_0 y"
  Demux5/3 -> Bus Creator/15  "Vhcl Fr1A_alpha_0 z"
  Demux4/1 -> Bus Creator/16  "Vhcl Fr1A_Tr2Fr0 00"
  Demux4/2 -> Bus Creator/17  "Vhcl Fr1A_Tr2Fr0 01"
  Demux4/3 -> Bus Creator/18  "Vhcl Fr1A_Tr2Fr0 02"
  Demux4/4 -> Bus Creator/19  "Vhcl Fr1A_Tr2Fr0 10"
  Demux4/5 -> Bus Creator/20  "Vhcl Fr1A_Tr2Fr0 11"
  Demux4/6 -> Bus Creator/21  "Vhcl Fr1A_Tr2Fr0 12"
  Demux4/7 -> Bus Creator/22  "Vhcl Fr1A_Tr2Fr0 20"
  Demux4/8 -> Bus Creator/23  "Vhcl Fr1A_Tr2Fr0 21"
  Demux4/9 -> Bus Creator/24  "Vhcl Fr1A_Tr2Fr0 22"
  Tr2Fr0/1 -> Demux4/1
  alpha_0/1 -> Demux5/1
  omega_0/1 -> Demux3/1
  a_0/1 -> Demux2/1
  v_0/1 -> Demux1/1
  t_0/1 -> Demux/1

== system UserVehicle_RTW/UserVehicle/CreateBus Vhcl.Fr1/Tr2Fr0 ==
  Car : Inport
  Bus Creator : BusCreator  Inputs=9
  Subsystem_00 : Subsystem
  Subsystem_01 : Subsystem
  Subsystem_02 : Subsystem
  Subsystem_10 : Subsystem
  Subsystem_11 : Subsystem
  Subsystem_12 : Subsystem
  Subsystem_20 : Subsystem
  Subsystem_21 : Subsystem
  Subsystem_22 : Subsystem
  sincos : Subsystem
  Tr2Fr0 : Outport  VectorParamsAs1DForOutWhenUnconnected=off
  wires:
  Subsystem_12/1(Tr2Fr1_12) -> Bus Creator/6  "Tr2Fr1_12"
  Subsystem_11/1(Tr2Fr1_11) -> Bus Creator/5  "Tr2Fr1_11"
  Subsystem_02/1(Tr2Fr1_02) -> Bus Creator/3  "Tr2Fr0_02"
  Subsystem_01/1(Tr2Fr1_01) -> Bus Creator/2  "Tr2Fr0_01"
  Subsystem_22/1(Tr2Fr1_22) -> Bus Creator/9  "Tr2Fr0_22"
  Subsystem_21/1(Tr2Fr1_21) -> Bus Creator/8  "Tr2Fr0_21"
  Subsystem_20/1(Tr2Fr1_20) -> Bus Creator/7  "Tr2Fr0_20"
  Subsystem_10/1(Tr2Fr1_10) -> Bus Creator/4  "Tr2Fr0_10"
  Subsystem_00/1(Tr2Fr1_00) -> Bus Creator/1  "Tr2Fr0_00"
  Bus Creator/1 -> Tr2Fr0/1
  sincos/1(sincos) -> Subsystem_02/1(sincos), Subsystem_01/1(sincos), Subsystem_00/1(sincos), Subsystem_12/1(sincos), Subsystem_22/1(sincos), Subsystem_21/1(sincos), Subsystem_20/1(sincos), Subsystem_11/1(sincos), Subsystem_10/1(sincos)
  Car/1 -> sincos/1(Car)

== system UserVehicle_RTW/UserVehicle/CreateBus Vhcl.Fr1/a_0 ==
  Car : Inport
  Tr2Fr0 : Inport  Port=2
  Add : Sum
  Add1 : Sum
  Add2 : Sum
  Bus Selector1 : BusSelector  OutputSignals=Car_a_1.Car_ax_1,Car_a_1.Car_ay_1
  Bus Selector2 : BusSelector  OutputSignals=Tr2Fr0_00,Tr2Fr0_01,Tr2Fr0_10,Tr2Fr1_11,Tr2Fr0_20,Tr2Fr0_21
  Mux1 : Mux  Inputs=3
  Product{,1..5} (6 alike) : Product  RndMeth=Zero
  a_0 : Outport  VectorParamsAs1DForOutWhenUnconnected=off
  wires:
  Bus Selector2/5 -> Product5/2  "<Tr2Fr0_20>"
  Bus Selector2/6 -> Product4/2  "<Tr2Fr0_21>"
  Add2/1 -> Mux1/3
  Product4/1 -> Add2/2
  Product5/1 -> Add2/1
  Bus Selector2/4 -> Product2/2  "<Tr2Fr1_11>"
  Bus Selector2/3 -> Product3/2  "<Tr2Fr0_10>"
  Add1/1 -> Mux1/2
  Bus Selector2/2 -> Product/2  "<Tr2Fr0_01>"
  Bus Selector2/1 -> Product1/2  "<Tr2Fr0_00>"
  Product2/1 -> Add1/2
  Product3/1 -> Add1/1
  Add/1 -> Mux1/1
  Product/1 -> Add/2
  Product1/1 -> Add/1
  Bus Selector1/1 -> Product5/1, Product3/1, Product1/1  "<Car_ax_1>"
  Bus Selector1/2 -> Product4/1, Product2/1, Product/1  "<Car_ay_1>"
  Tr2Fr0/1 -> Bus Selector2/1
  Car/1 -> Bus Selector1/1
  Mux1/1 -> a_0/1

== system UserVehicle_RTW/UserVehicle/CreateBus Vhcl.Fr1/t_0 ==
  Car : Inport
  Bus Selector : BusSelector  OutputSignals=Car_t_0.Car_tx_0,Car_t_0.Car_ty_0,Road_Fr1_z
  Mux : Mux  Inputs=3
  t_0 : Outport  VectorParamsAs1DForOutWhenUnconnected=off
  wires:
  Mux/1 -> t_0/1
  Car/1 -> Bus Selector/1
  Bus Selector/3 -> Mux/3  "<Road_Fr1_z>"
  Bus Selector/2 -> Mux/2  "<Car_ty_0>"
  Bus Selector/1 -> Mux/1  "<Car_tx_0>"

== system UserVehicle_RTW/UserVehicle/CreateBus Vhcl.Fr1/v_0 ==
  Car : Inport
  Tr2Fr0 : Inport  Port=2
  Bus Selector1 : BusSelector  OutputSignals=Car_v_1.Car_vx_1
  Bus Selector2 : BusSelector  OutputSignals=Tr2Fr0_00,Tr2Fr0_10,Tr2Fr0_20
  Mux1 : Mux  Inputs=3
  Product : Product  RndMeth=Zero
  Product1 : Product  RndMeth=Zero
  Product2 : Product  RndMeth=Zero
  v_0 : Outport  VectorParamsAs1DForOutWhenUnconnected=off
  wires:
  Product2/1 -> Mux1/3
  Product1/1 -> Mux1/2
  Product/1 -> Mux1/1
  Bus Selector1/1 -> Product2/1, Product1/1, Product/1  "<Car_vx_1>"
  Bus Selector2/3 -> Product2/2  "<Tr2Fr0_20>"
  Bus Selector2/2 -> Product1/2  "<Tr2Fr0_10>"
  Bus Selector2/1 -> Product/2  "<Tr2Fr0_00>"
  Tr2Fr0/1 -> Bus Selector2/1
  Mux1/1 -> v_0/1
  Car/1 -> Bus Selector1/1

== system UserVehicle_RTW/UserVehicle/Query Road CoG/Subsystem ==
  xyz : Inport
  Dist : Inport  Port=2
  Side : Inport  Port=3
  Enable : EnablePort
  IPGRoad5 : CarMaker4SL/IPGRoad5  xname=IPGRoad  xevalmode=RouteEval XY_S  xconsiderbumps=off  xusepath=off  xwithcurve=off  xabort=on
      settings: SourceProductName=CarMaker4SL
  Mux : Mux  Inputs=2
  Terminator : Terminator
  Tire : Outport  VectorParamsAs1DForOutWhenUnconnected=off
  wires:
  IPGRoad5/1 -> Terminator/1
  Dist/1 -> Mux/1
  Side/1 -> Mux/2
  Mux/1 -> IPGRoad5/1
  xyz/1 -> IPGRoad5/2
  IPGRoad5/2 -> Tire/1

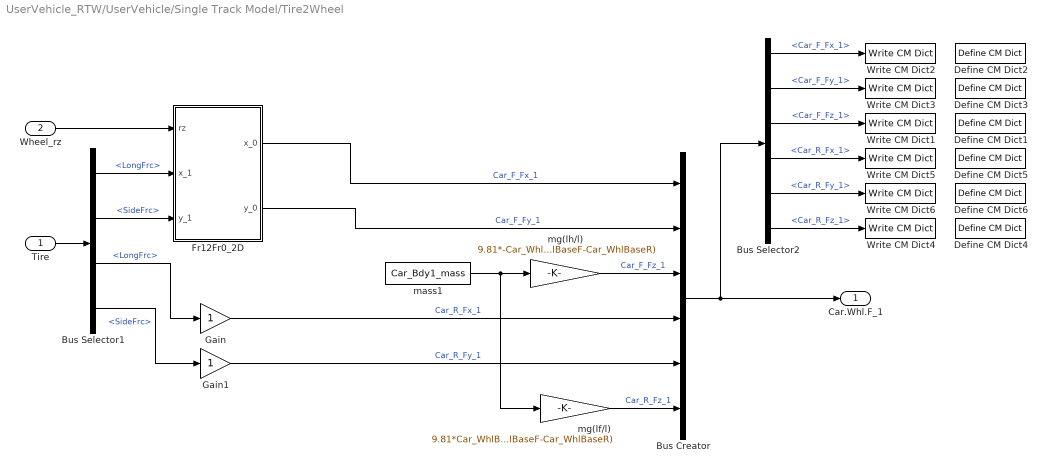
== system UserVehicle_RTW/UserVehicle/Single Track Model/Tire2Wheel ==
  Tire : Inport
  Wheel_rz : Inport  Port=2
  Bus Creator : BusCreator  Inputs=6
  Bus Selector1 : BusSelector  OutputSignals=Car_Tire_F.LongFrc,Car_Tire_F.SideFrc,Car_Tire_R.LongFrc,Car_Tire_R.SideFrc
  Bus Selector2 : BusSelector  OutputSignals=Car_F_Fx_1,Car_F_Fy_1,Car_F_Fz_1,Car_R_Fx_1,Car_R_Fy_1,Car_R_Fz_1
  Define CM Dict1 : CarMaker4SL/Define CM Dict  xname=Car.F.Fz_1  xunit=N  xmono=off  xtype=Double4  xdvaplace=None  xnstates=0  xfirststate=0  xinitial=0
  Define CM Dict2 : CarMaker4SL/Define CM Dict  xname=Car.F.Fx_1  xunit=N  xmono=off  xtype=Double4  xdvaplace=None  xnstates=0  xfirststate=0  xinitial=0
  Define CM Dict3 : CarMaker4SL/Define CM Dict  xname=Car.F.Fy_1  xunit=N  xmono=off  xtype=Double4  xdvaplace=None  xnstates=0  xfirststate=0  xinitial=0
  Define CM Dict4 : CarMaker4SL/Define CM Dict  xname=Car.R.Fz_1  xunit=N  xmono=off  xtype=Double4  xdvaplace=None  xnstates=0  xfirststate=0  xinitial=0
  Define CM Dict5 : CarMaker4SL/Define CM Dict  xname=Car.R.Fx_1  xunit=N  xmono=off  xtype=Double4  xdvaplace=None  xnstates=0  xfirststate=0  xinitial=0
  Define CM Dict6 : CarMaker4SL/Define CM Dict  xname=Car.R.Fy_1  xunit=N  xmono=off  xtype=Double4  xdvaplace=None  xnstates=0  xfirststate=0  xinitial=0
  Fr12Fr0_2D : Subsystem
  Gain : Gain
  Gain1 : Gain
  Write CM Dict1 : CarMaker4SL/Write CM Dict  xname=Car.F.Fz_1  xsync=off
  Write CM Dict2 : CarMaker4SL/Write CM Dict  xname=Car.F.Fx_1  xsync=off
  Write CM Dict3 : CarMaker4SL/Write CM Dict  xname=Car.F.Fy_1  xsync=off
  Write CM Dict4 : CarMaker4SL/Write CM Dict  xname=Car.R.Fz_1  xsync=off
  Write CM Dict5 : CarMaker4SL/Write CM Dict  xname=Car.R.Fx_1  xsync=off
  Write CM Dict6 : CarMaker4SL/Write CM Dict  xname=Car.R.Fy_1  xsync=off
  mass1 : Constant  Value=Car_Bdy1_mass
  mg(lf/l) : Gain  Gain=9.81*Car_WhlBaseF/(Car_WhlBaseF-Car_WhlBaseR)  SaturateOnIntegerOverflow=on  OutDataTypeStr=Inherit: Same as input  ParamDataTypeStr=Inherit: Same as input
  mg(lh/l) : Gain  Gain=9.81*-Car_WhlBaseR/(Car_WhlBaseF-Car_WhlBaseR)  SaturateOnIntegerOverflow=on  OutDataTypeStr=Inherit: Same as input  ParamDataTypeStr=Inherit: Same as input
  Car.Whl.F_1 : Outport  VectorParamsAs1DForOutWhenUnconnected=off
  wires:
  Fr12Fr0_2D/1(x_0) -> Bus Creator/1  "Car_F_Fx_1"
  Bus Selector2/6 -> Write CM Dict4/1  "<Car_R_Fz_1>"
  Bus Selector2/5 -> Write CM Dict6/1  "<Car_R_Fy_1>"
  Bus Selector2/4 -> Write CM Dict5/1  "<Car_R_Fx_1>"
  Bus Selector2/3 -> Write CM Dict1/1  "<Car_F_Fz_1>"
  Bus Selector2/2 -> Write CM Dict3/1  "<Car_F_Fy_1>"
  Bus Selector2/1 -> Write CM Dict2/1  "<Car_F_Fx_1>"
  mg(lf/l)/1 -> Bus Creator/6  "Car_R_Fz_1"
  mg(lh/l)/1 -> Bus Creator/3  "Car_F_Fz_1"
  mass1/1 -> mg(lf/l)/1, mg(lh/l)/1
  Wheel_rz/1 -> Fr12Fr0_2D/1(rz)
  Fr12Fr0_2D/2(y_0) -> Bus Creator/2  "Car_F_Fy_1"
  Gain1/1 -> Bus Creator/5  "Car_R_Fy_1"
  Gain/1 -> Bus Creator/4  "Car_R_Fx_1"
  Bus Selector1/4 -> Gain1/1  "<SideFrc>"
  Bus Selector1/3 -> Gain/1  "<LongFrc>"
  Bus Selector1/2 -> Fr12Fr0_2D/3(y_1)  "<SideFrc>"
  Bus Selector1/1 -> Fr12Fr0_2D/2(x_1)  "<LongFrc>"
  Bus Creator/1 -> Bus Selector2/1, Car.Whl.F_1/1
  Tire/1 -> Bus Selector1/1

== system UserVehicle_RTW/UserVehicle/Single Track Model/sideslip angle ==
  Car_a_1 : Inport
  Car_v_1 : Inport  Port=2
  Yaw : Inport  Port=3
  "  " : Product  InputSameDT=on  SaturateOnIntegerOverflow=on  OutDataTypeStr=Inherit: Same as first input
  Bus Creator : BusCreator  Inputs=2
  Bus Selector1 : BusSelector  OutputSignals=Yawp
  Bus Selector2 : BusSelector  OutputSignals=Car_ay_1,Car_ax_1
  Bus Selector3 : BusSelector  OutputSignals=Car_vx_1
  Define CM Dict : CarMaker4SL/Define CM Dict  xname=Car.SideSlipAngVel  xunit=rad/s  xmono=off  xtype=Double4  xdvaplace=None  xnstates=0  xfirststate=0  xinitial=0
  Define CM Dict1 : CarMaker4SL/Define CM Dict  xname=Car.SideSlipAng  xunit=rad  xmono=off  xtype=Double4  xdvaplace=None  xnstates=0  xfirststate=0  xinitial=0
  Subsystem : Subsystem
  Sum2 : Sum  Inputs=+-  InputSameDT=on  SaturateOnIntegerOverflow=on  OutDataTypeStr=Inherit: Same as first input
  Write CM Dict : CarMaker4SL/Write CM Dict  xname=Car.SideSlipAngVel  xsync=off
  Write CM Dict1 : CarMaker4SL/Write CM Dict  xname=Car.SideSlipAng  xsync=off
  beta_dot * dt : Integrator  ExternalReset=level
  beta : Outport  VectorParamsAs1DForOutWhenUnconnected=off
  wires:
  Subsystem/1(Out1) -> Write CM Dict/1, Bus Creator/2, beta_dot * dt/1  "betap"
  beta_dot * dt/1 -> Write CM Dict1/1, Bus Creator/1, "  "/2  "beta"
  Bus Selector3/1 -> Subsystem/2(v)  "<Car_vx_1>"
  Bus Selector2/2 -> "  "/1  "<Car_ax_1>"
  Bus Selector2/1 -> Sum2/1  "<Car_ay_1>"
  Car_a_1/1 -> Bus Selector2/1
  Bus Creator/1 -> beta/1
  Bus Selector1/1 -> Subsystem/1(vYaw)  "<Yawp>"
  Yaw/1 -> Bus Selector1/1
  Car_v_1/1 -> Bus Selector3/1
  Sum2/1 -> Subsystem/3(In3)
  "  "/1 -> Sum2/2
  [TRStart] -> beta_dot * dt/2

== system UserVehicle_RTW/UserVehicle/Single Track Model/steer kinematic ==
  In1 : Inport
  Bus Selector4 : BusSelector  OutputSignals=VhclCtrl Steering Ang
  "Steering_i " : Gain  Gain=1/Car_Steering_i  SaturateOnIntegerOverflow=on  OutDataTypeStr=Inherit: Same as input  ParamDataTypeStr=Inherit: Same as input
  Car.Whl.F.rz : Outport  VectorParamsAs1DForOutWhenUnconnected=off
  wires:
  "Steering_i "/1 -> Car.Whl.F.rz/1
  In1/1 -> Bus Selector4/1
  Bus Selector4/1 -> "Steering_i "/1  "<VhclCtrl Steering Ang>"
